simulink model "drone2DStep_without_controller"  (R2014a)
settings: Solver=ode45  StartTime=0.0  StopTime=10.0  RelTol=1e-3
settings Model: Creator=ravik  LastModifiedBy=ravik

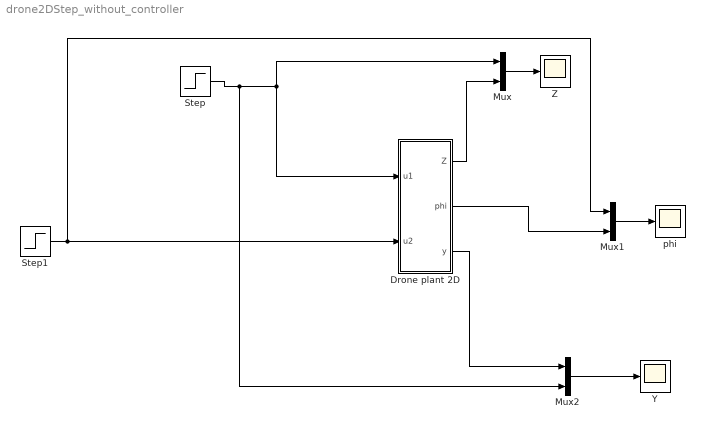
== system drone2DStep_without_controller ==
  Drone plant 2D : Subsystem
  Mux : Mux  Inputs=2
  Mux1 : Mux  Inputs=2
  Mux2 : Mux  Inputs=2
  Step : Step  SampleTime=0
  Step1 : Step  SampleTime=0
  Y : Scope
      settings: SaveName=ScopeData2
  Z : Scope
  phi : Scope
  wires:
  Step/1 -> Mux2/2, Drone plant 2D/1(u1), Mux/1
  Drone plant 2D/1(Z) -> Mux/2
  Drone plant 2D/2(phi) -> Mux1/2
  Drone plant 2D/3(y) -> Mux2/1
  Mux/1 -> Z/1
  Mux1/1 -> phi/1
  Mux2/1 -> Y/1
  Step1/1 -> Mux1/1, Drone plant 2D/2(u2)

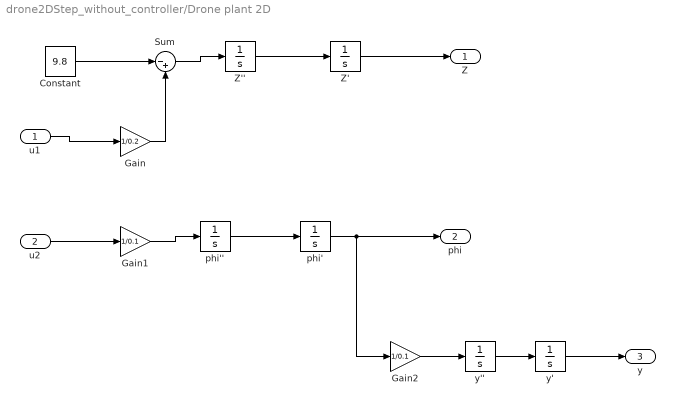
== system drone2DStep_without_controller/Drone plant 2D ==
  u1 : Inport
  u2 : Inport  Port=2
  Constant : Constant  Value=9.8
  Gain : Gain  Gain=1/0.2
  Gain1 : Gain  Gain=1/0.1
  Gain2 : Gain  Gain=1/0.1
  Sum : Sum  Inputs=|-+
  Z' : Integrator
  Z'' : Integrator
  phi' : Integrator
  phi'' : Integrator
  y' : Integrator
  y'' : Integrator
  Z : Outport
  phi : Outport  Port=2
  y : Outport  Port=3
  wires:
  Sum/1 -> Z''/1
  phi'/1 -> phi/1, Gain2/1
  Gain/1 -> Sum/2
  Z'/1 -> Z/1
  phi''/1 -> phi'/1
  Z''/1 -> Z'/1
  y'/1 -> y/1
  Gain1/1 -> phi''/1
  u1/1 -> Gain/1
  Constant/1 -> Sum/1
  Gain2/1 -> y''/1
  y''/1 -> y'/1
  u2/1 -> Gain1/1
